simulink model "Simulation_Vehicule"  (R2018a)
settings: Solver=VariableStepAuto  StartTime=0.0  StopTime=3600  RelTol=1e-3
libraries: Vehicule x1, ForcesExterieures x1, Conducteur x1
settings Model: Creator=Thomas  LastModifiedBy=thomas.moser
settings SolverCC: ZeroCrossAlgorithm=Adaptive
settings DebuggingCC: MaxConsecutiveZCsMsg=none  IgnoredZcDiagnostic=none

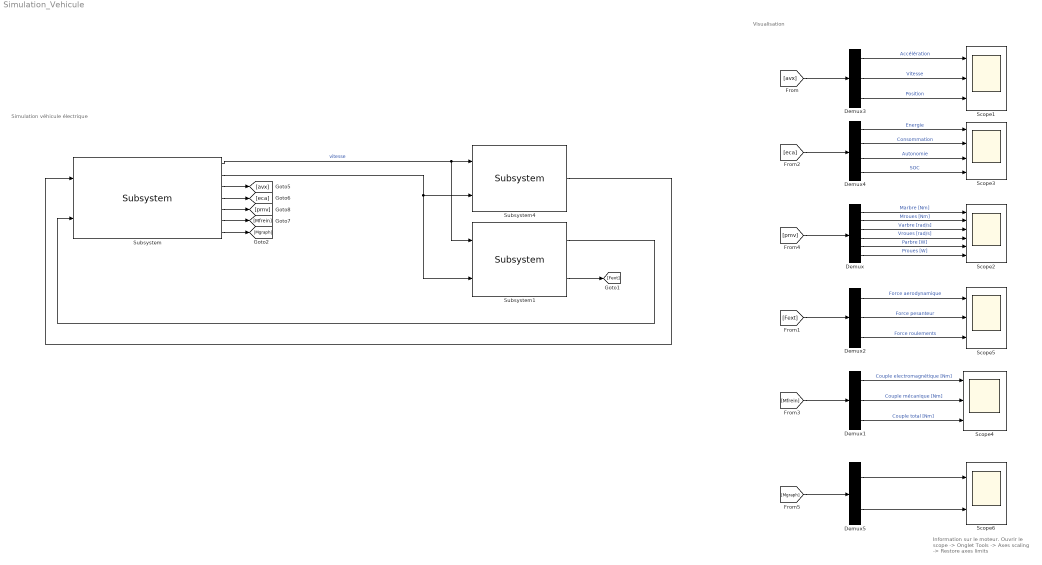
== system Simulation_Vehicule ==
  note: Information sur le moteur.
      | Ouvrir le scope -> Onglet Tools ->
      | Axes scaling -> Restore axes limits
  note: Visualisation
  note: Simulation véhicule électrique
  Demux : Demux  Outputs=6
  Demux1 : Demux  Outputs=3
  Demux2 : Demux  Outputs=3
  Demux3 : Demux  Outputs=3
  Demux4 : Demux
  Demux5 : Demux  Outputs=2
  Scope1 : Scope  NumInputPorts=3
  Scope2 : Scope  NumInputPorts=6
  Scope3 : Scope  NumInputPorts=4
  Scope4 : Scope  NumInputPorts=3
  Scope5 : Scope  NumInputPorts=3
  Scope6 : Scope  NumInputPorts=2
  Subsystem : Vehicule/Subsystem  m=2250  mp=80  rr=0.33  s=1  cx=0.5  crr=0.015  mlimit=660  alimit=3  Vmin=25/3.6  Vmax=250/3.6  r=9.73  nr=0.9  nm=0.89  Pmax=310380  Mmax=660  nc=0.89  cb=98  soc=99  tempExt=25  nbrCycle=0
  Subsystem1 : ForcesExterieures/Subsystem  rho=1.225  g=9.81
  Subsystem4 : Conducteur/Subsystem  SystemSampleTime=-1
      link override Compare To Constant: const=dist_tot_int
  wires:
  Demux/1 -> Scope2/1  "Marbre [Nm]"
  Demux/2 -> Scope2/2  "Mroues [Nm]"
  Demux/3 -> Scope2/3  "Varbre [rad/s]"
  Demux/4 -> Scope2/4  "Vroues [rad/s]"
  Demux/5 -> Scope2/5  "Parbre [W]"
  Demux/6 -> Scope2/6  "Proues [W]"
  Subsystem4/1 -> Subsystem/1
  Demux1/1 -> Scope4/1  "Couple electromagnétique [Nm]"
  Demux1/2 -> Scope4/2  "Couple mécanique [Nm]"
  Demux1/3 -> Scope4/3  "Couple total [Nm]"
  [avx] -> Demux3/1
  Demux3/1 -> Scope1/1  "Accélération"
  Demux3/2 -> Scope1/2  "Vitesse"
  Demux3/3 -> Scope1/3  "Position"
  Subsystem/1 -> Subsystem1/1, Subsystem4/1  "vitesse"
  Subsystem1/2 -> [Fext]
  Demux2/1 -> Scope5/1  "Force aerodynamique"
  Demux2/2 -> Scope5/2  "Force pesanteur"
  Demux2/3 -> Scope5/3  "Force roulements"
  [Fext] -> Demux2/1
  Demux4/3 -> Scope3/3  "Autonomie"
  [eca] -> Demux4/1
  Demux4/1 -> Scope3/1  "Energie"
  Demux4/2 -> Scope3/2  "Consommation"
  Demux4/4 -> Scope3/4  "SOC"
  Subsystem/2 -> Subsystem1/2, Subsystem4/2
  [Mfrein] -> Demux1/1
  [pmv] -> Demux/1
  Subsystem1/1 -> Subsystem/2
  Subsystem/6 -> [Mfrein]
  Subsystem/5 -> [pmv]
  Subsystem/4 -> [eca]
  Subsystem/3 -> [avx]
  Subsystem/7 -> [Mgraph]
  [Mgraph] -> Demux5/1
  Demux5/1 -> Scope6/1
  Demux5/2 -> Scope6/2
